simulink model "Comparison_Systems_Analog"  (R2017a)
settings: Solver=ode4  StartTime=0.0  StopTime=0.5  FixedStep=Tsim  RelTol=1e-3
values from neighbouring files (symbols this model uses):
  a = 25    [Stetup_HIL.m]
  K = 20    [Stetup_HIL.m]
  T = 1/Fs    (= 0.002)    [Stetup_HIL.m]
settings Model: Creator=tac29  LastModifiedBy=Merc

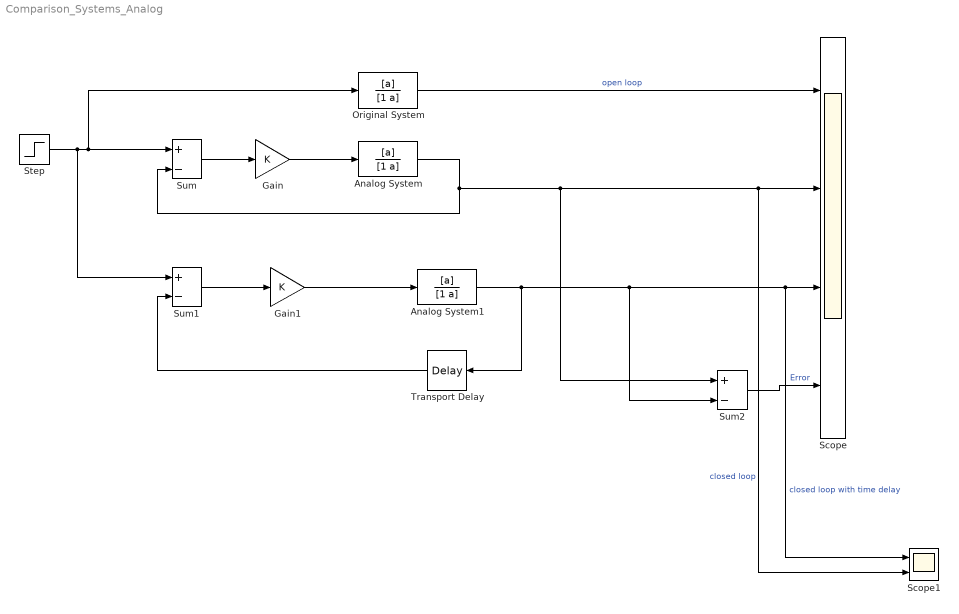
== system Comparison_Systems_Analog ==
  Analog System : TransferFcn  Numerator=[a]  Denominator=[1 a]
  Analog System1 : TransferFcn  Numerator=[a]  Denominator=[1 a]
  Gain : Gain  Gain=K
  Gain1 : Gain  Gain=K
  "Original System " : TransferFcn  Numerator=[a]  Denominator=[1 a]
  Scope : Scope  NumInputPorts=4
  Scope1 : Scope  NumInputPorts=2
  Step : Step  Time=.1  SampleTime=0
  Sum : Sum  Inputs=+-
  Sum1 : Sum  Inputs=+-
  Sum2 : Sum  Inputs=+-
  Transport Delay : TransportDelay  DelayTime=T
  wires:
  Analog System/1 -> Sum/2, Sum2/1, Scope1/2, Scope/2  "closed loop"
  Sum/1 -> Gain/1
  Gain/1 -> Analog System/1
  "Original System "/1 -> Scope/1  "open loop"
  Step/1 -> Sum1/1, "Original System "/1, Sum/1
  Sum1/1 -> Gain1/1
  Gain1/1 -> Analog System1/1
  Analog System1/1 -> Transport Delay/1, Sum2/2, Scope1/1, Scope/3  "closed loop with time delay"
  Transport Delay/1 -> Sum1/2
  Sum2/1 -> Scope/4  "Error"
